simulink model "chap2_7sim"  (R2016b)
settings: Solver=ode45  StartTime=0.0  StopTime=RunTime  FixedStep=0.001  MaxStep=0.005  RelTol=1e-3  EnableMultiTasking=on
settings Model: Creator=Masoud  LastModifiedBy=Hafez
settings SolverCC: InitialStep=0.005
settings DataIOCC: LimitDataPoints=on  SaveFormat=Array
settings OptimizationCC: LifeSpan=inf
settings DebuggingCC: SFUnexpectedBacktrackingDiag=warning  SFNoUnconditionalDefaultTransitionDiag=warning  SFExecutionAtInitializationDiag=none
settings HardwareCC: ProdBitPerPointer=32  ProdBitPerSizeT=32  ProdBitPerPtrDiffT=32  ProdLargestAtomicFloat=None  ProdIntDivRoundTo=Undefined  ProdEndianess=Unspecified  ProdWordSize=32  ProdHWDeviceType=32-bit Generic
settings ModelReferenceCC: PropagateSignalLabelsOutOfModel=off
settings GRTTargetCC: TargetLangStandard=C89/C90 (ANSI)  GeneratePreprocessorConditionals=Disable all
settings ConfigComp: CovMetricSettings=dw  CovHtmlReporting=on  CovSaveCumulativeToWorkspaceVar=on  CovSaveSingleToWorkspaceVar=on  CovExternalEMLEnable=off

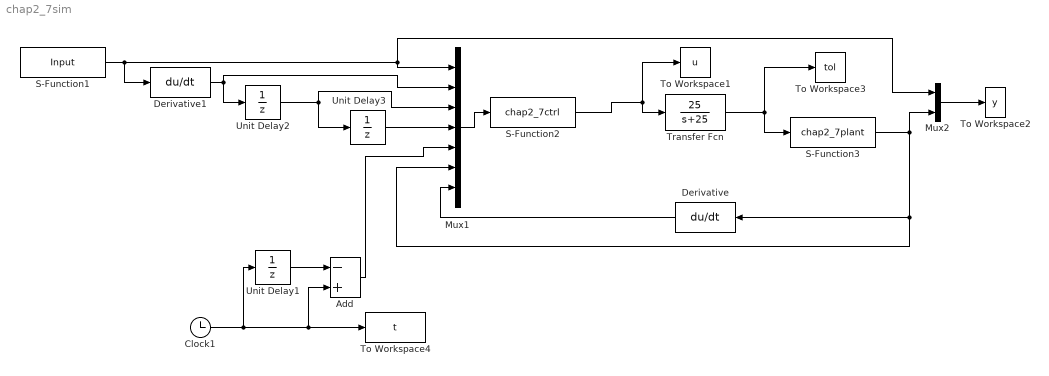
== system chap2_7sim ==
  Add : Sum  Inputs=-+
  Clock1 : Clock
  Derivative : Derivative
  Derivative1 : Derivative
  Mux1 : Mux  Inputs=7
  Mux2 : Mux  Inputs=2
  S-Function1 : S-Function  FunctionName=Input  SFunctionModules='Input'  SFunctionDeploymentMode=off  EnableBusSupport=off
  S-Function2 : S-Function  FunctionName=chap2_7ctrl  SFunctionModules='chap2_7ctrl'  SFunctionDeploymentMode=off  EnableBusSupport=off
  S-Function3 : S-Function  FunctionName=chap2_7plant  SFunctionModules='chap2_7plant'  SFunctionDeploymentMode=off  EnableBusSupport=off
  To Workspace1 : ToWorkspace  VariableName=u  SampleTime=-1
  To Workspace2 : ToWorkspace  VariableName=y  SampleTime=-1
  To Workspace3 : ToWorkspace  VariableName=tol  SampleTime=-1
  To Workspace4 : ToWorkspace  VariableName=t  SampleTime=-1
  Transfer Fcn : TransferFcn  Numerator=[25]  Denominator=[1 25]
  Unit Delay1 : UnitDelay  SampleTime=-1
  Unit Delay2 : UnitDelay  SampleTime=-1
  Unit Delay3 : UnitDelay  SampleTime=-1
  wires:
  Mux1/1 -> S-Function2/1
  Mux2/1 -> To Workspace2/1
  S-Function3/1 -> Mux1/6, Derivative/1, Mux2/2
  Derivative/1 -> Mux1/7
  Transfer Fcn/1 -> S-Function3/1, To Workspace3/1
  S-Function1/1 -> Mux2/1, Mux1/1, Derivative1/1
  Derivative1/1 -> Unit Delay2/1, Mux1/2
  Unit Delay2/1 -> Unit Delay3/1, Mux1/3
  Clock1/1 -> Unit Delay1/1, Add/2, To Workspace4/1
  Unit Delay1/1 -> Add/1
  Add/1 -> Mux1/5
  Unit Delay3/1 -> Mux1/4
  S-Function2/1 -> Transfer Fcn/1, To Workspace1/1
